simulink model "Buck_Simulink"  (R2023a)
settings: Solver=VariableStepAuto  StartTime=0.0  StopTime=1  RelTol=1e-3
values from neighbouring files (symbols this model uses):
  C = 10e-6    (= 1e-05)    [Buck_ED.m]
  L = 2e-3    (= 0.002)    [Buck_ED.m]
  R = 10    [Buck_ED.m]
  Uin = 32    [Buck_ED.m]
settings Model: Creator=fermo  LastModifiedBy=mluser
settings OptimizationCC: ReuseModelBlockBuffer=off

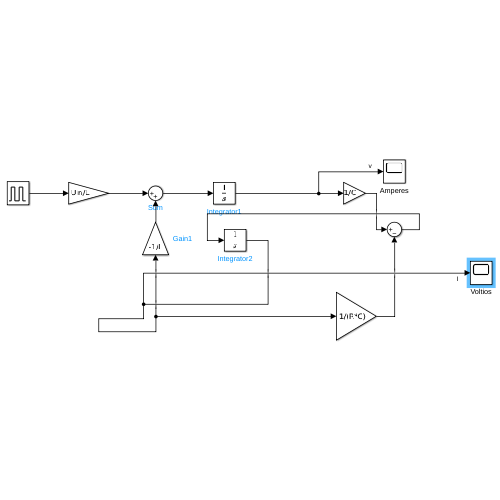
[thumbnail: Simulink's stored preview of the top-level diagram]
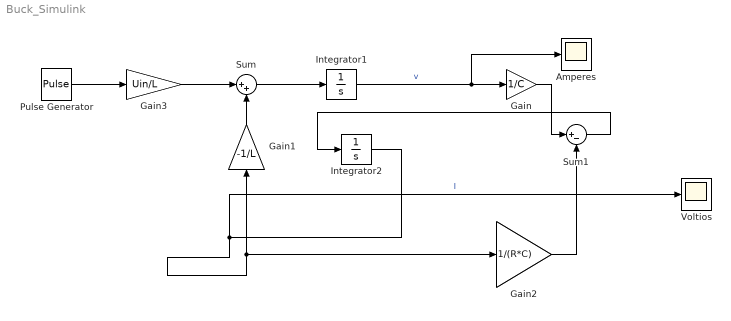
== system Buck_Simulink ==
  Amperes : Scope
  Gain : Gain  Gain=1/C
  Gain1 : Gain  Gain=-1/L
  Gain2 : Gain  Gain=1/(R*C)
  Gain3 : Gain  Gain=Uin/L
  Integrator1 : Integrator
  Integrator2 : Integrator
  Pulse Generator : DiscretePulseGenerator  PulseType=Time based  Period=0.0001  PulseWidth=40
  Sum : Sum  Inputs=|++
  Sum1 : Sum  Inputs=|+-
  Voltios : Scope
  wires:
  Pulse Generator/1 -> Gain3/1
  Gain3/1 -> Sum/1
  Gain1/1 -> Sum/2
  Integrator2/1 -> Gain1/1, Gain2/1, Voltios/1  "I"
  Integrator1/1 -> Amperes/1, Gain/1  "v"
  Gain2/1 -> Sum1/2
  Gain/1 -> Sum1/1
  Sum1/1 -> Integrator2/1
  Sum/1 -> Integrator1/1
